simulink model "halfly_controlled_three_phase_bridge_rectifier"  (R2022a)
settings: Solver=VariableStepAuto  StartTime=0.0  StopTime=0.04  RelTol=1e-3
libraries: spsVoltageMeasurementLib x6, spsDiodeLib x3, spsDetailedThyristorLib x3, spsACVoltageSourceLib x3, spsCurrentMeasurementLib x2, spsSeriesRLCBranchLib x1, spsGroundLib x1, spspowerguiLib x1
settings Model: Creator=alireza  LastModifiedBy=P.O.M.G
settings SolverCC: AlgebraicLoopSolver=TrustRegion
settings DataIOCC: ReturnWorkspaceOutputs=off
settings OptimizationCC: LifeSpan=inf
settings DebuggingCC: UnconnectedInputMsg=warning  UnconnectedOutputMsg=warning  UnconnectedLineMsg=warning  SFExecutionAtInitializationDiag=none  SFMachineParentedDataDiag=warning  ArithmeticOperatorsInVariantConditions=warning
settings SFSimCC: CustomCodeUndefinedFunction=UseInterfaceOnly
settings CodeAppCC: StateflowObjectComments=on

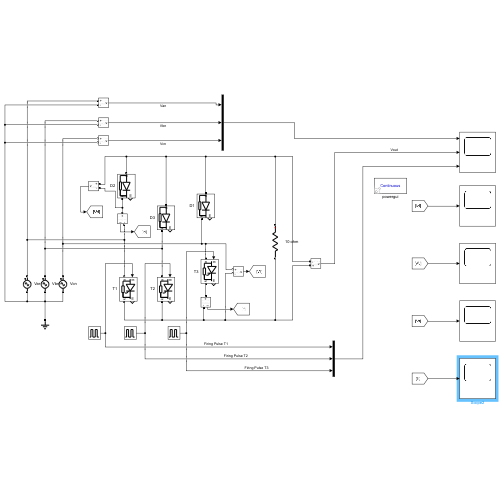
[thumbnail: Simulink's stored preview of the top-level diagram]
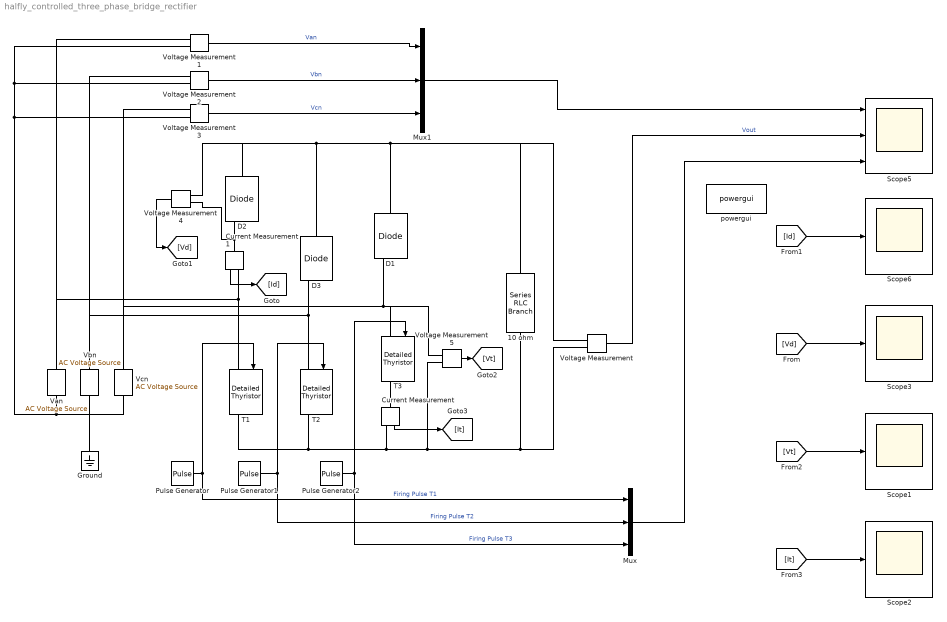
== system halfly_controlled_three_phase_bridge_rectifier ==
  10 ohm : spsSeriesRLCBranchLib/Series RLC Branch  LConnTagsString=__new0  RConnTagsString=__new0  BranchType=R  Resistance=10  Inductance=1e-3  SetiL0=off  InitialCurrent=0  Capacitance=1e-6  Setx0=off  InitialVoltage=0  Measurements=None
  Current Measurement : spsCurrentMeasurementLib/Current Measurement  PhasorSimulation=off  OutputType=Complex  PSBequivalent=0
  Current Measurement1 : spsCurrentMeasurementLib/Current Measurement  PhasorSimulation=off  OutputType=Complex  PSBequivalent=0
  D1 : spsDiodeLib/Diode  Ron=0.001  Lon=0  Vf=0.8  IC=0  UseSnubber=0  Rs=500  Cs=250e-9  Measurements=on
  D2 : spsDiodeLib/Diode  Ron=0.001  Lon=0  Vf=0.8  IC=0  UseSnubber=0  Rs=500  Cs=250e-9  Measurements=on
  D3 : spsDiodeLib/Diode  Ron=0.001  Lon=0  Vf=0.8  IC=0  UseSnubber=0  Rs=500  Cs=250e-9  Measurements=on
  Ground : spsGroundLib/Ground  LConnTagsString=a
  Mux : Mux  Inputs=3
  Mux1 : Mux  Inputs=3
  Pulse Generator : DiscretePulseGenerator  PulseType=Time based  Period=0.02  PulseWidth=5  PhaseDelay=0.005
  Pulse Generator1 : DiscretePulseGenerator  PulseType=Time based  Period=0.02  PulseWidth=5  PhaseDelay=0.01167
  Pulse Generator2 : DiscretePulseGenerator  PulseType=Time based  Period=0.02  PulseWidth=5  PhaseDelay=0.01833
  Scope{1..3,6} (4 alike) : Scope
  Scope5 : Scope  NumInputPorts=3
  T1 : spsDetailedThyristorLib/Detailed Thyristor  Ron=0.001  Lon=1e-3  Vf=0.8  IL=0.1  Tq=100e-6  IC=0  Rs=500  Cs=250e-9  Measurements=on
      settings: SourceProductBaseCode=PS
  T2 : spsDetailedThyristorLib/Detailed Thyristor  Ron=0.001  Lon=1e-3  Vf=0.8  IL=0.1  Tq=100e-6  IC=0  Rs=500  Cs=250e-9  Measurements=on
      settings: SourceProductBaseCode=PS
  T3 : spsDetailedThyristorLib/Detailed Thyristor  Ron=0.001  Lon=1e-3  Vf=0.8  IL=0.1  Tq=100e-6  IC=0  Rs=500  Cs=250e-9  Measurements=on
      settings: SourceProductBaseCode=PS
  Van : spsACVoltageSourceLib/AC Voltage Source  Amplitude=308  Phase=0  Frequency=50  SampleTime=0  Measurements=None  BusType=swing  Pref=10e3  Qref=0  Qmin=-inf  Qmax=+inf
  Vbn : spsACVoltageSourceLib/AC Voltage Source  Amplitude=308  Phase=120  Frequency=50  SampleTime=0  Measurements=None  BusType=swing  Pref=10e3  Qref=0  Qmin=-inf  Qmax=+inf
  Vcn : spsACVoltageSourceLib/AC Voltage Source  Amplitude=308  Phase=240  Frequency=50  SampleTime=0  Measurements=None  BusType=swing  Pref=10e3  Qref=0  Qmin=-inf  Qmax=+inf
  Voltage Measurement{,1..5} (6 alike) : spsVoltageMeasurementLib/Voltage Measurement  PhasorSimulation=off  OutputType=Complex  PSBequivalent=0
  powergui : spspowerguiLib/powergui  Priority=1  SimulationMode=Continuous  SampleTime=50e-6  frequency=60  Iterations=50  frequencyindice=50  Pbase=100e6  ErrMax=1e-4  UnitsV=kV  UnitsW=MW  buscounter=0  FunctionMessages=off  echomessages=off  EnableUseOfTLC=off  CurrentSourceSwitches=off  DisableSnubberDevices=off  DisableRonSwitches=off  DisableVfSwitches=off  DisplayEquations=off  AutomaticDiscreteSolvers=off  SolverType=Tustin/Backward Euler (TBE)  Interpol=off  ExternalGateDelay=off  methode=off  Ts=100  x0status=blocks  SPID=on  SwTol=0  HookPort=off  NonlinearTolerance=1e-4  nMaxIteration=100  ContinueOnMaxIteration=off  RestoreLinks=warning  ResistiveCurrentMeasurement=off  Frange=[0:2:500]  Ylog=off  Xlog=on  ShowGrid=off  save=off  variable=ZData  structure=0  ZoomFFT=off  StartTime=0.0  cycles=1  DisplayStyle=1  fundamental=60  FreqAxis=off  MaxFrequency=1000  frequencyindicesteady=1  RmsSteady=1  display=off
  wires:
  Pulse Generator/1 -> Mux/1, T1/1  "Firing Pulse T1"
  Pulse Generator1/1 -> T2/1, Mux/2  "Firing Pulse T2"
  Pulse Generator2/1 -> T3/1, Mux/3  "Firing Pulse T3"
  Voltage Measurement1/1 -> Mux1/1  "Van"
  Voltage Measurement2/1 -> Mux1/2  "Vbn"
  Voltage Measurement3/1 -> Mux1/3  "Vcn"
  Mux1/1 -> Scope5/1
  Voltage Measurement/1 -> Scope5/2  "Vout"
  Mux/1 -> Scope5/3
  [Vd] -> Scope3/1
  [Id] -> Scope6/1
  Current Measurement1/1 -> [Id]
  Voltage Measurement4/1 -> [Vd]
  Voltage Measurement5/1 -> [Vt]
  Current Measurement/1 -> [It]
  [Vt] -> Scope1/1
  [It] -> Scope2/1
  connections:
  Voltage Measurement1/LConn2 -- Voltage Measurement3/LConn2 -- Van/LConn1 -- Vcn/LConn1 -- Ground/LConn1 -- Vbn/LConn1 -- Voltage Measurement2/LConn2
  Voltage Measurement1/LConn1 -- Van/RConn1 -- Current Measurement1/RConn1 -- T1/LConn1
  Voltage Measurement2/LConn1 -- Vbn/RConn1 -- T2/LConn1 -- D3/RConn1
  D1/RConn1 -- Voltage Measurement5/LConn1 -- T3/LConn1 -- Vcn/RConn1 -- Voltage Measurement3/LConn1
  10 ohm/RConn1 -- Voltage Measurement5/LConn2 -- Current Measurement/RConn1 -- T2/RConn1 -- T1/RConn1 -- Voltage Measurement/LConn1
  D3/LConn1 -- D2/LConn1 -- Voltage Measurement4/LConn1 -- 10 ohm/LConn1 -- Voltage Measurement/LConn2 -- D1/LConn1
  Current Measurement/LConn1 -- T3/RConn1
  D2/RConn1 -- Voltage Measurement4/LConn2 -- Current Measurement1/LConn1
